simulink model "angle_motor"  (R2021b)
settings: Solver=FixedStepDiscrete  StartTime=0.0  StopTime=inf  FixedStep=0.0005  RelTol=1e-3
model workspace (MAT data in the model file):
  data = 30
  data2 = -30
libraries: simulink x9, IFR_StackLiteDualDrive_SimulinkLib x4
settings Model: Creator=ysl  LastModifiedBy=ysl
settings OptimizationCC: DefaultParameterBehavior=Inlined  EnhancedBackFolding=on  PassReuseOutputArgsAs=Individual arguments  ZeroExternalMemoryAtStartup=off  ZeroInternalMemoryAtStartup=off  OptimizeBlockOrder=speed  DifferentSizesBufferReuse=on  OptimizationCustomize=off  EfficientTunableParamExpr=on
settings DebuggingCC: ParameterTunabilityLossMsg=error
settings SFSimCC: MATLABDynamicMemAlloc=off
settings RTWCC: Description=IFR StackLite-DualDrive Base on stm32f405RGT6  SystemTargetFile=stacklite_dualdrive.tlc  TemplateMakefile=stacklite_dualdrive.tmf  GenerateReport=on
settings CodeAppCC: ForceParamTrailComments=on  IgnoreCustomStorageClasses=off  OperatorAnnotations=on  SimulinkDataObjDesc=on  SFDataObjDesc=on  InsertBlockDesc=on
settings STFCustomTargetCC: TargetLangStandard=C99 (ISO)  MultiwordLength=256  ParMdlRefBuildCompliant=on  CompOptLevelCompliant=on  CombineOutputUpdateFcns=on  ERTCustomFileBanners=on  SupportContinuousTime=off  SupportNonInlinedSFcns=off  RemoveResetFunc=on  MATLABClassNameForMDSCustomization=Simulink.SoftwareTarget.ERTCustomization  CPPClassGenCompliant=on  GRTInterface=off  SystemTargetFile=stacklite_dualdrive.tlc
settings ERTTargetCC: TargetLangStandard=C99 (ISO)  ConcurrentExecutionCompliant=off  ModelStepFunctionPrototypeControlCompliant=off  UseToolchainInfoCompliant=off  InlinedParameterPlacement=NonHierarchical  ERTCustomFileTemplate=example_file_process.tlc

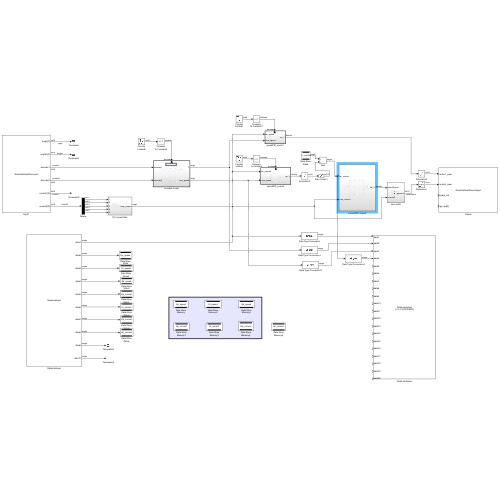
[thumbnail: Simulink's stored preview of the top-level diagram]
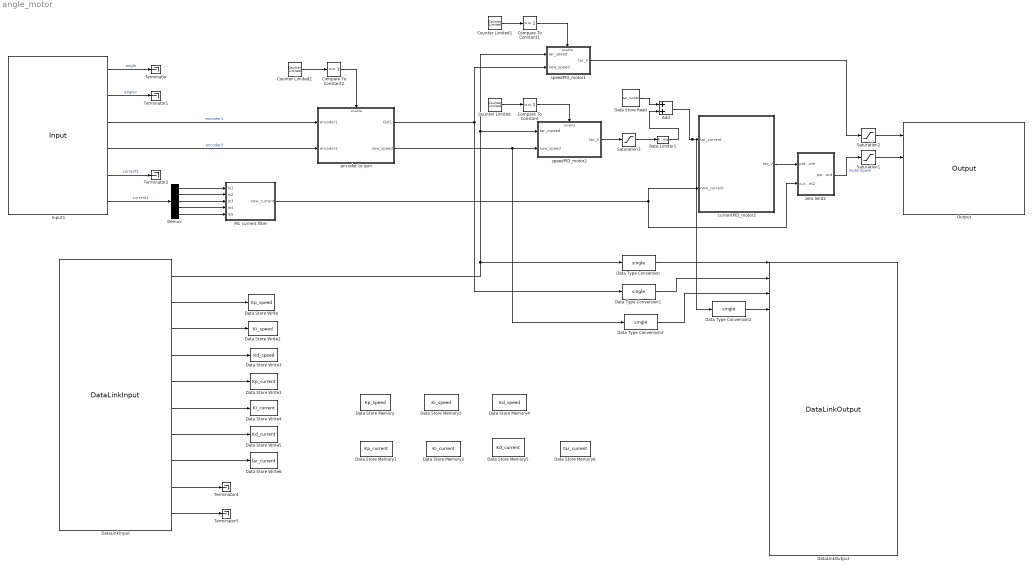
== system angle_motor ==
  Add : Sum
  Compare To Constant : simulink/Logic and Bit Operations/Compare To Constant  relop===  const=1  OutDataTypeStr=boolean
  Compare To Constant1 : simulink/Logic and Bit Operations/Compare To Constant  relop===  const=1  OutDataTypeStr=boolean
  Compare To Constant2 : simulink/Logic and Bit Operations/Compare To Constant  relop===  const=1  OutDataTypeStr=boolean
  Counter Limited : simulink/Sources/Counter Limited  uplimit=1  tsamp=-1
  Counter Limited1 : simulink/Sources/Counter Limited  uplimit=1  tsamp=-1
  Counter Limited2 : simulink/Sources/Counter Limited  uplimit=1  tsamp=-1
  Data Store Memory : DataStoreMemory  DataStoreName=Kp_speed  ReadBeforeWriteMsg=warning  WriteAfterWriteMsg=warning  WriteAfterReadMsg=warning  ShowAdditionalParam=off
  Data Store Memory1 : DataStoreMemory  DataStoreName=Kp_current  ReadBeforeWriteMsg=warning  WriteAfterWriteMsg=warning  WriteAfterReadMsg=warning  ShowAdditionalParam=off
  Data Store Memory2 : DataStoreMemory  DataStoreName=Ki_speed  ReadBeforeWriteMsg=warning  WriteAfterWriteMsg=warning  WriteAfterReadMsg=warning  ShowAdditionalParam=off
  Data Store Memory3 : DataStoreMemory  DataStoreName=Ki_current  ReadBeforeWriteMsg=warning  WriteAfterWriteMsg=warning  WriteAfterReadMsg=warning  ShowAdditionalParam=off
  Data Store Memory4 : DataStoreMemory  DataStoreName=Kd_speed  ReadBeforeWriteMsg=warning  WriteAfterWriteMsg=warning  WriteAfterReadMsg=warning  ShowAdditionalParam=off
  Data Store Memory5 : DataStoreMemory  DataStoreName=Kd_current  ReadBeforeWriteMsg=warning  WriteAfterWriteMsg=warning  WriteAfterReadMsg=warning  ShowAdditionalParam=off
  Data Store Memory6 : DataStoreMemory  DataStoreName=tar_current  ReadBeforeWriteMsg=warning  WriteAfterWriteMsg=warning  WriteAfterReadMsg=warning  ShowAdditionalParam=off
  Data Store Read : DataStoreRead  DataStoreName=tar_current  IndexOptions=Index vector (dialog)  Indices=1  OutputSizes=1
  Data Store Write : DataStoreWrite  DataStoreName=Kp_speed  IndexOptions=Index vector (dialog)  Indices=1  OutputSizes=1
  Data Store Write1 : DataStoreWrite  DataStoreName=Kp_current  IndexOptions=Index vector (dialog)  Indices=1  OutputSizes=1
  Data Store Write2 : DataStoreWrite  DataStoreName=Ki_speed  IndexOptions=Index vector (dialog)  Indices=1  OutputSizes=1
  Data Store Write3 : DataStoreWrite  DataStoreName=Kd_speed  IndexOptions=Index vector (dialog)  Indices=1  OutputSizes=1
  Data Store Write4 : DataStoreWrite  DataStoreName=Ki_current  IndexOptions=Index vector (dialog)  Indices=1  OutputSizes=1
  Data Store Write5 : DataStoreWrite  DataStoreName=Kd_current  IndexOptions=Index vector (dialog)  Indices=1  OutputSizes=1
  Data Store Write6 : DataStoreWrite  DataStoreName=tar_current  IndexOptions=Index vector (dialog)  Indices=1  OutputSizes=1
  Data Type Conversion{,1..3} (4 alike) : DataTypeConversion  OutDataTypeStr=single
  DataLinkInput : IFR_StackLiteDualDrive_SimulinkLib/DataLinkInput
      settings: SourceProductName=IFR_StackLiteDualDrive_SimulinkLib_V1.0
  DataLinkOutput : IFR_StackLiteDualDrive_SimulinkLib/DataLinkOutput  id='BalanceUnname'  key='IFR00'
      settings: SourceProductName=IFR_StackLiteDualDrive_SimulinkLib_V1.0
  Demux : Demux  Outputs=5
  Input1 : IFR_StackLiteDualDrive_SimulinkLib/Input  Priority=0
      settings: SourceProductName=IFR_StackLiteDualDrive_SimulinkLib_V1.0
  M1 current filter : Subsystem
  Output : IFR_StackLiteDualDrive_SimulinkLib/Output  Priority=255
      settings: SourceProductName=IFR_StackLiteDualDrive_SimulinkLib_V1.0
  Rate Limiter1 : RateLimiter  RisingSlewLimit=10000  FallingSlewLimit=-10000  SampleTimeMode=inherited
  Saturation1 : Saturate  UpperLimit=4200  LowerLimit=-4200  OutDataTypeStr=int16
  Saturation2 : Saturate  UpperLimit=4200  LowerLimit=-4200  OutDataTypeStr=int16
  Saturation3 : Saturate  UpperLimit=2048  LowerLimit=-2048  OutDataTypeStr=int16
  Terminator{,1..2,4..5} (5 alike) : Terminator
  currentPID_motor2 : Subsystem
  encoder to rpm : Subsystem
  speedPID_motor1 : Subsystem
  speedPID_motor2 : Subsystem
  zero limit2 : Subsystem
  wires:
  Input1/6 -> Demux/1  "current1"
  Demux/1 -> M1 current filter/1(In1)
  Demux/2 -> M1 current filter/2(In2)
  Demux/3 -> M1 current filter/3(In3)
  Demux/4 -> M1 current filter/4(In4)
  Demux/5 -> M1 current filter/5(In5)
  DataLinkInput/2 -> Data Store Write/1
  DataLinkInput/3 -> Data Store Write2/1
  DataLinkInput/4 -> Data Store Write3/1
  DataLinkInput/5 -> Data Store Write1/1
  DataLinkInput/6 -> Data Store Write4/1
  DataLinkInput/7 -> Data Store Write5/1
  Input1/1 -> Terminator/1  "angle"
  Input1/2 -> Terminator1/1  "anglev"
  DataLinkInput/9 -> Terminator4/1
  DataLinkInput/10 -> Terminator5/1
  Data Type Conversion/1 -> DataLinkOutput/1
  Data Type Conversion1/1 -> DataLinkOutput/2
  Input1/5 -> Terminator2/1  "current1"
  speedPID_motor2/1(tar_V) -> Saturation3/1
  Counter Limited/1 -> Compare To Constant/1
  Compare To Constant/1 -> speedPID_motor2/Enable
  DataLinkInput/1 -> speedPID_motor2/1(tar_cspeed), speedPID_motor1/1(tar_speed), Data Type Conversion/1
  speedPID_motor1/1(tar_V) -> Saturation2/1
  Counter Limited1/1 -> Compare To Constant1/1
  Compare To Constant1/1 -> speedPID_motor1/Enable
  Saturation3/1 -> Rate Limiter1/1
  M1 current filter/1(now_current) -> zero limit2/2(current2), currentPID_motor2/2(now_current)
  Saturation1/1 -> Output/2
  encoder to rpm/1(Out1) -> Data Type Conversion1/1, speedPID_motor1/2(now_speed)
  Input1/3 -> encoder to rpm/1(encoder1)  "encoder1"
  Input1/4 -> encoder to rpm/2(encoder2)  "encoder2"
  Counter Limited2/1 -> Compare To Constant2/1
  Compare To Constant2/1 -> encoder to rpm/Enable
  encoder to rpm/2(now_speed) -> Data Type Conversion3/1, speedPID_motor2/2(now_speed)
  currentPID_motor2/1(tar_V) -> zero limit2/1(pidout2pwm)
  zero limit2/1(pwmout) -> Saturation1/1  "motor2pwm"
  Saturation2/1 -> Output/1
  Data Type Conversion3/1 -> DataLinkOutput/3
  DataLinkInput/8 -> Data Store Write6/1
  Data Store Read/1 -> Add/1
  Rate Limiter1/1 -> Add/2
  Add/1 -> currentPID_motor2/1(tar_current), Data Type Conversion2/1
  Data Type Conversion2/1 -> DataLinkOutput/4

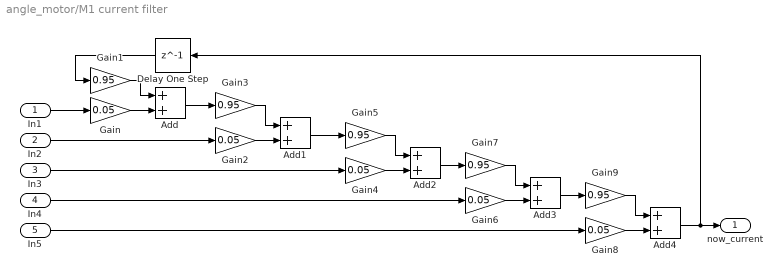
== system angle_motor/M1 current filter ==
  In1 : Inport
  In2 : Inport  Port=2
  In3 : Inport  Port=3
  In4 : Inport  Port=4
  In5 : Inport  Port=5
  Add{,1..4} (5 alike) : Sum
  Delay One Step : Delay  DelayLength=1
  Gain{,2,4,6,8} (5 alike) : Gain  Gain=0.05  OutDataTypeStr=single
  Gain{1,3,5,7,9} (5 alike) : Gain  Gain=0.95  OutDataTypeStr=single
  now_current : Outport
  wires:
  Add4/1 -> now_current/1, Delay One Step/1
  In5/1 -> Gain8/1
  Add3/1 -> Gain9/1
  Gain9/1 -> Add4/1
  Gain8/1 -> Add4/2
  In4/1 -> Gain6/1
  Add2/1 -> Gain7/1
  Gain7/1 -> Add3/1
  Gain6/1 -> Add3/2
  In3/1 -> Gain4/1
  Add1/1 -> Gain5/1
  Gain5/1 -> Add2/1
  Gain4/1 -> Add2/2
  In2/1 -> Gain2/1
  Gain3/1 -> Add1/1
  Gain2/1 -> Add1/2
  Add/1 -> Gain3/1
  Gain1/1 -> Add/1
  Delay One Step/1 -> Gain1/1
  Gain/1 -> Add/2
  In1/1 -> Gain/1

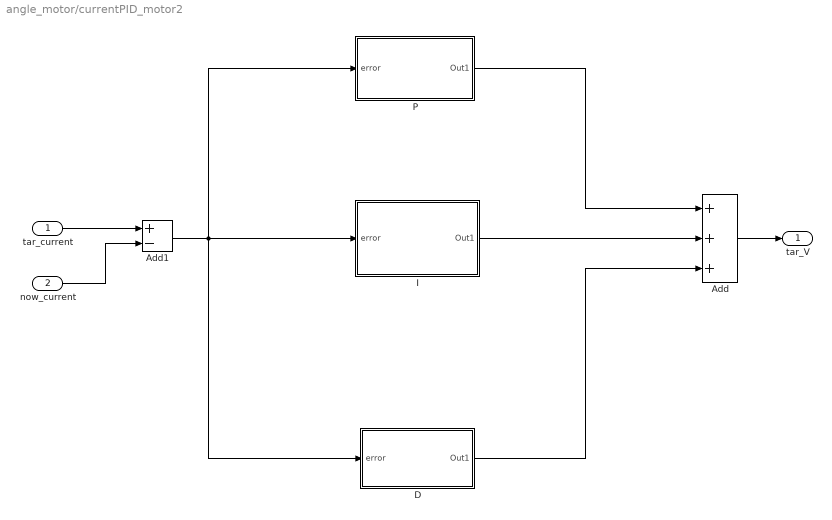
== system angle_motor/currentPID_motor2 ==
  tar_current : Inport
  now_current : Inport  Port=2
  Add : Sum  Inputs=+++  OutDataTypeStr=double
  Add1 : Sum  Inputs=+-
  D : Subsystem
  I : Subsystem
  P : Subsystem
  tar_V : Outport
  wires:
  now_current/1 -> Add1/2
  Add/1 -> tar_V/1
  tar_current/1 -> Add1/1
  Add1/1 -> D/1(error), I/1(error), P/1(error)
  P/1(Out1) -> Add/1
  I/1(Out1) -> Add/2
  D/1(Out1) -> Add/3

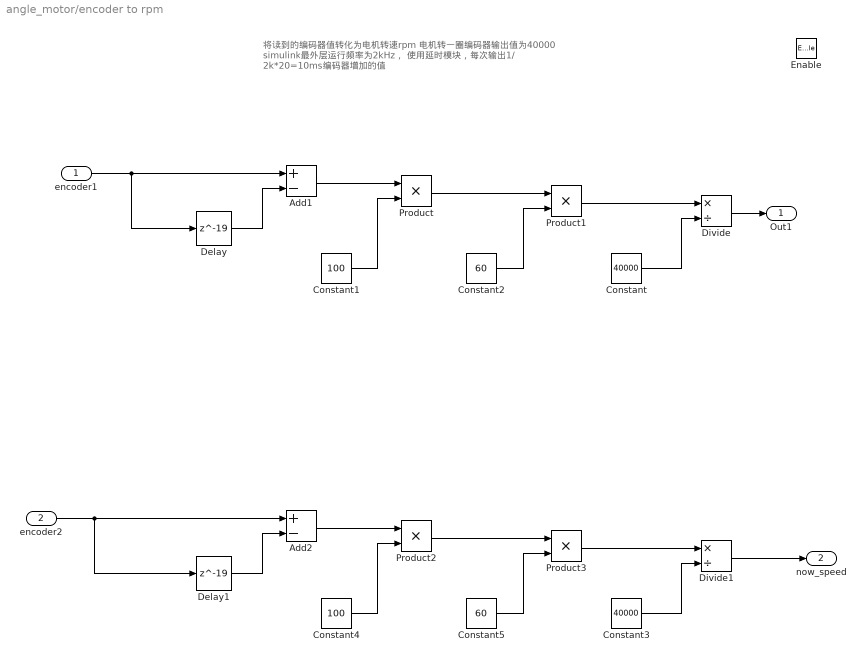
== system angle_motor/encoder to rpm ==
  note: 将读到的编码器值转化为电机转速rpm
      | 电机转一圈编码器输出值为40000
      | simulink最外层运行频率为2kHz，
      | 使用延时模块，每次输出1/ 2k*20=10ms编码器增加的值
  encoder1 : Inport
  encoder2 : Inport  Port=2
  Enable : EnablePort
  Add1 : Sum  Inputs=+-
  Add2 : Sum  Inputs=+-
  Constant : Constant  Value=40000  OutDataTypeStr=single
  Constant1 : Constant  Value=100  OutDataTypeStr=single
  Constant2 : Constant  Value=60  OutDataTypeStr=single
  Constant3 : Constant  Value=40000  OutDataTypeStr=single
  Constant4 : Constant  Value=100  OutDataTypeStr=single
  Constant5 : Constant  Value=60  OutDataTypeStr=single
  Delay : Delay  DelayLength=19
  Delay1 : Delay  DelayLength=19
  Divide : Product  Inputs=*/  OutDataTypeStr=single
  Divide1 : Product  Inputs=*/  OutDataTypeStr=single
  Product{,1..3} (4 alike) : Product  OutDataTypeStr=single
  Out1 : Outport
  now_speed : Outport  Port=2
  wires:
  Product1/1 -> Divide/1
  Product/1 -> Product1/1
  Constant/1 -> Divide/2
  encoder1/1 -> Add1/1, Delay/1
  Add2/1 -> Product2/1
  Delay1/1 -> Add2/2
  encoder2/1 -> Add2/1, Delay1/1
  Constant1/1 -> Product/2
  Add1/1 -> Product/1
  Constant2/1 -> Product1/2
  Delay/1 -> Add1/2
  Divide1/1 -> now_speed/1
  Product2/1 -> Product3/1
  Constant4/1 -> Product2/2
  Product3/1 -> Divide1/1
  Constant5/1 -> Product3/2
  Divide/1 -> Out1/1
  Constant3/1 -> Divide1/2

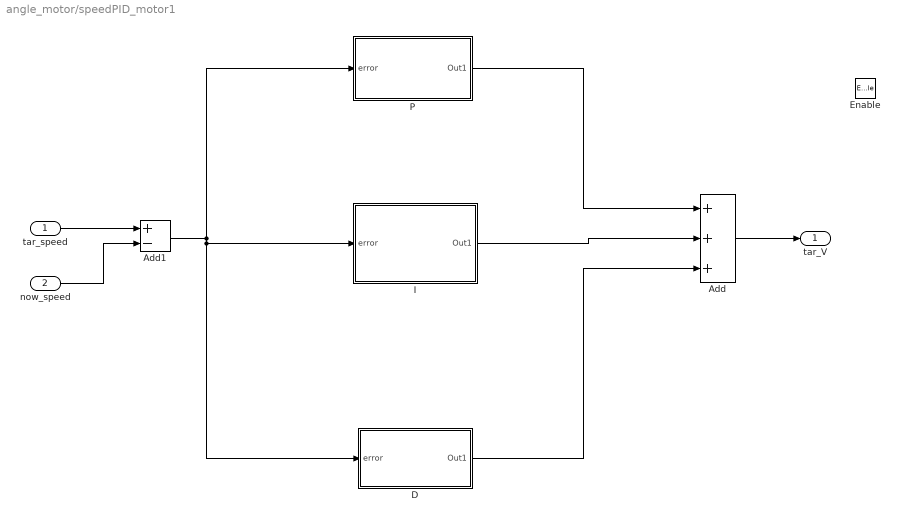
== system angle_motor/speedPID_motor1 ==
  tar_speed : Inport
  now_speed : Inport  Port=2
  Enable : EnablePort
  Add : Sum  Inputs=+++  OutDataTypeStr=double
  Add1 : Sum  Inputs=+-
  D : Subsystem
  I : Subsystem
  P : Subsystem
  tar_V : Outport
  wires:
  D/1(Out1) -> Add/3
  tar_speed/1 -> Add1/1
  P/1(Out1) -> Add/1
  Add/1 -> tar_V/1
  Add1/1 -> D/1(error), I/1(error), P/1(error)
  now_speed/1 -> Add1/2
  I/1(Out1) -> Add/2

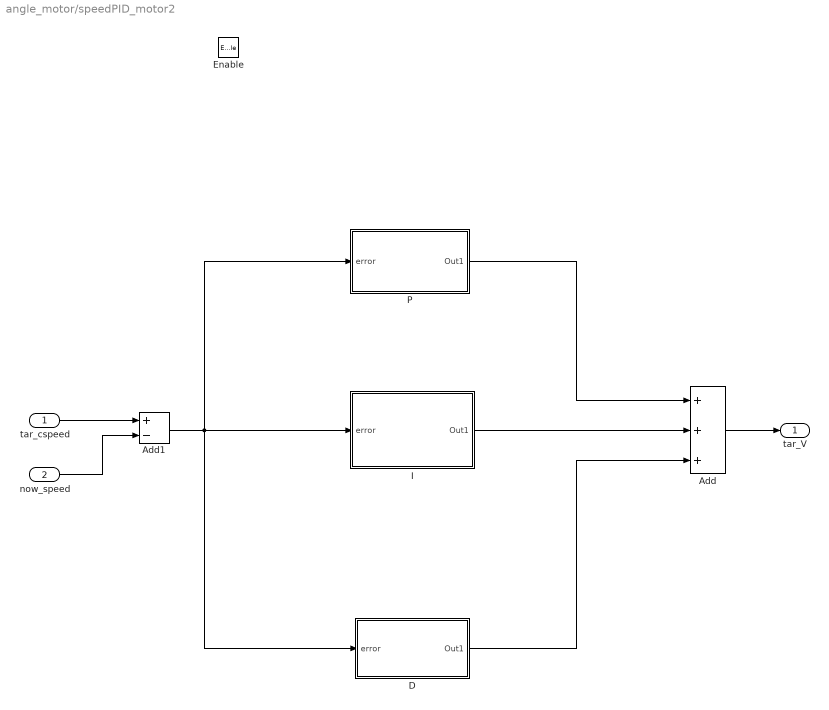
== system angle_motor/speedPID_motor2 ==
  tar_cspeed : Inport
  now_speed : Inport  Port=2
  Enable : EnablePort
  Add : Sum  Inputs=+++  OutDataTypeStr=double
  Add1 : Sum  Inputs=+-
  D : Subsystem
  I : Subsystem
  P : Subsystem
  tar_V : Outport
  wires:
  Add/1 -> tar_V/1
  now_speed/1 -> Add1/2
  I/1(Out1) -> Add/2
  P/1(Out1) -> Add/1
  Add1/1 -> D/1(error), I/1(error), P/1(error)
  D/1(Out1) -> Add/3
  tar_cspeed/1 -> Add1/1

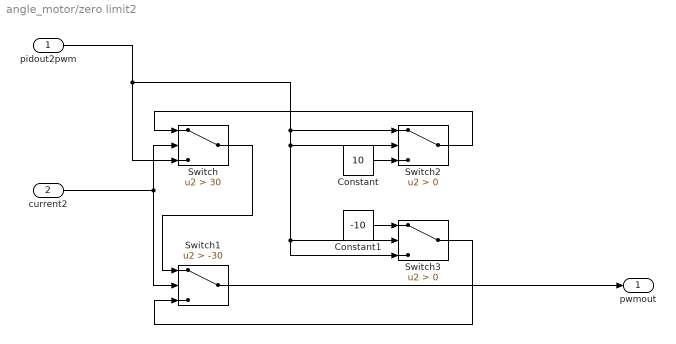
== system angle_motor/zero limit2 ==
  pidout2pwm : Inport
  current2 : Inport  Port=2
  Constant : Constant  Value=10  OutDataTypeStr=int16
  Constant1 : Constant  Value=-10  OutDataTypeStr=int16
  Switch : Switch  Criteria=u2 > Threshold  Threshold=30  OutDataTypeStr=int16
  Switch1 : Switch  Criteria=u2 > Threshold  Threshold=-30  OutDataTypeStr=int16
  Switch2 : Switch  Criteria=u2 > Threshold  OutDataTypeStr=int16
  Switch3 : Switch  Criteria=u2 > Threshold  OutDataTypeStr=int16
  pwmout : Outport
  wires:
  Switch1/1 -> pwmout/1
  Switch2/1 -> Switch/1
  Switch3/1 -> Switch1/3
  Switch/1 -> Switch1/1
  Constant/1 -> Switch2/3
  pidout2pwm/1 -> Switch2/2, Switch3/2, Switch3/3, Switch2/1, Switch/3
  current2/1 -> Switch1/2, Switch/2
  Constant1/1 -> Switch3/1

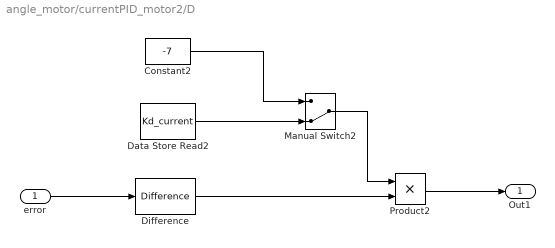
== system angle_motor/currentPID_motor2/D ==
  error : Inport
  Constant2 : Constant  Value=-7
  Data Store Read2 : DataStoreRead  DataStoreName=Kd_current  IndexOptions=Index vector (dialog)  Indices=1  OutputSizes=1
  Difference : simulink/Discrete/Difference  ICPrevInput=0.0  OutMin=[]  OutMax=[]  OutDataType=fixdt(1, 16)  OutScaling=2^-10  DoSatur=off
  Manual Switch2 : ManualSwitch  CurrentSetting=0
  Product2 : Product
  Out1 : Outport
  wires:
  Difference/1 -> Product2/2
  Product2/1 -> Out1/1
  Data Store Read2/1 -> Manual Switch2/2
  Manual Switch2/1 -> Product2/1
  Constant2/1 -> Manual Switch2/1
  error/1 -> Difference/1

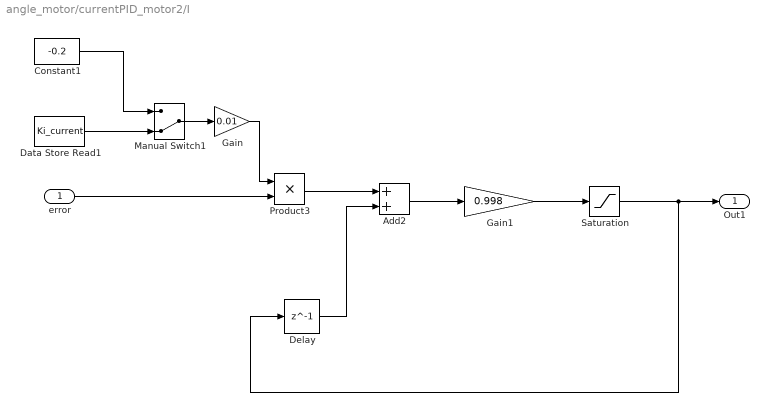
== system angle_motor/currentPID_motor2/I ==
  error : Inport
  Add2 : Sum
  Constant1 : Constant  Value=-0.2
  Data Store Read1 : DataStoreRead  DataStoreName=Ki_current  IndexOptions=Index vector (dialog)  Indices=1  OutputSizes=1
  Delay : Delay  DelayLength=1
  Gain : Gain  Gain=0.01
  Gain1 : Gain  Gain=0.998
  Manual Switch1 : ManualSwitch  CurrentSetting=0
  Product3 : Product  OutDataTypeStr=single
  Saturation : Saturate  UpperLimit=2000  LowerLimit=-2000
  Out1 : Outport
  wires:
  Delay/1 -> Add2/2
  Gain/1 -> Product3/1
  Add2/1 -> Gain1/1
  Constant1/1 -> Manual Switch1/1
  Manual Switch1/1 -> Gain/1
  Data Store Read1/1 -> Manual Switch1/2
  Product3/1 -> Add2/1
  error/1 -> Product3/2
  Gain1/1 -> Saturation/1
  Saturation/1 -> Delay/1, Out1/1

== system angle_motor/currentPID_motor2/P ==
  error : Inport
  Constant : Constant  Value=-2
  Data Store Read : DataStoreRead  DataStoreName=Kp_current  IndexOptions=Index vector (dialog)  Indices=1  OutputSizes=1
  Manual Switch : ManualSwitch  CurrentSetting=0
  Product : Product
  Out1 : Outport
  wires:
  error/1 -> Product/2
  Manual Switch/1 -> Product/1
  Data Store Read/1 -> Manual Switch/2
  Constant/1 -> Manual Switch/1
  Product/1 -> Out1/1

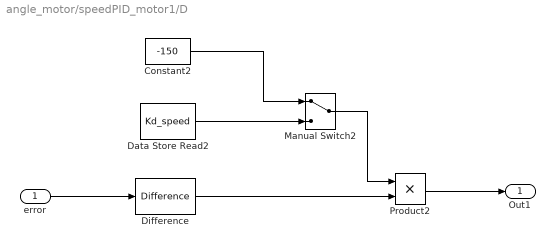
== system angle_motor/speedPID_motor1/D ==
  error : Inport
  Constant2 : Constant  Value=-150
  Data Store Read2 : DataStoreRead  DataStoreName=Kd_speed  IndexOptions=Index vector (dialog)  Indices=1  OutputSizes=1
  Difference : simulink/Discrete/Difference  ICPrevInput=0.0  OutMin=[]  OutMax=[]  OutDataType=fixdt(1, 16)  OutScaling=2^-10  DoSatur=off
  Manual Switch2 : ManualSwitch
  Product2 : Product
  Out1 : Outport
  wires:
  Difference/1 -> Product2/2
  Product2/1 -> Out1/1
  Data Store Read2/1 -> Manual Switch2/2
  Manual Switch2/1 -> Product2/1
  Constant2/1 -> Manual Switch2/1
  error/1 -> Difference/1

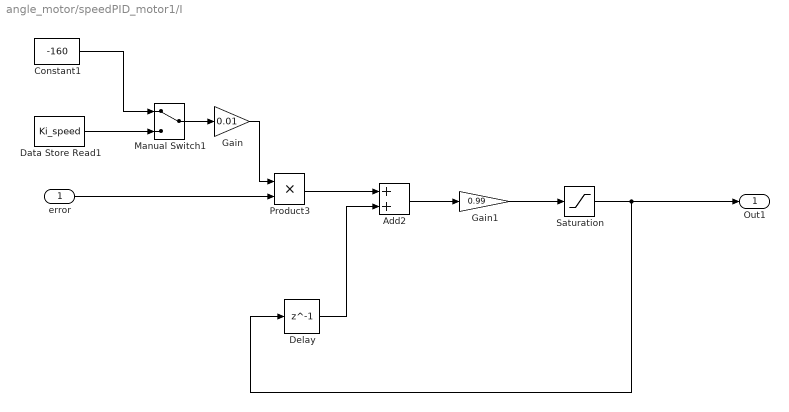
== system angle_motor/speedPID_motor1/I ==
  error : Inport
  Add2 : Sum
  Constant1 : Constant  Value=-160
  Data Store Read1 : DataStoreRead  DataStoreName=Ki_speed  IndexOptions=Index vector (dialog)  Indices=1  OutputSizes=1
  Delay : Delay  DelayLength=1
  Gain : Gain  Gain=0.01
  Gain1 : Gain  Gain=0.99
  Manual Switch1 : ManualSwitch
  Product3 : Product  OutDataTypeStr=single
  Saturation : Saturate  UpperLimit=600  LowerLimit=-600
  Out1 : Outport
  wires:
  Delay/1 -> Add2/2
  Gain/1 -> Product3/1
  Add2/1 -> Gain1/1
  Constant1/1 -> Manual Switch1/1
  Manual Switch1/1 -> Gain/1
  Data Store Read1/1 -> Manual Switch1/2
  Gain1/1 -> Saturation/1
  Product3/1 -> Add2/1
  error/1 -> Product3/2
  Saturation/1 -> Out1/1, Delay/1

== system angle_motor/speedPID_motor1/P ==
  error : Inport
  Constant : Constant  Value=-40
  Data Store Read : DataStoreRead  DataStoreName=Kp_speed  IndexOptions=Index vector (dialog)  Indices=1  OutputSizes=1
  Manual Switch : ManualSwitch
  Product : Product
  Out1 : Outport
  wires:
  error/1 -> Product/2
  Manual Switch/1 -> Product/1
  Data Store Read/1 -> Manual Switch/2
  Constant/1 -> Manual Switch/1
  Product/1 -> Out1/1

== system angle_motor/speedPID_motor2/D ==
  error : Inport
  Constant2 : Constant  Value=55
  Data Store Read2 : DataStoreRead  DataStoreName=Kd_speed  IndexOptions=Index vector (dialog)  Indices=1  OutputSizes=1
  Difference : simulink/Discrete/Difference  ICPrevInput=0.0  OutMin=[]  OutMax=[]  OutDataType=fixdt(1, 16)  OutScaling=2^-10  DoSatur=off
  Manual Switch2 : ManualSwitch  CurrentSetting=0
  Product2 : Product
  Out1 : Outport
  wires:
  Difference/1 -> Product2/2
  Product2/1 -> Out1/1
  Data Store Read2/1 -> Manual Switch2/2
  Manual Switch2/1 -> Product2/1
  Constant2/1 -> Manual Switch2/1
  error/1 -> Difference/1

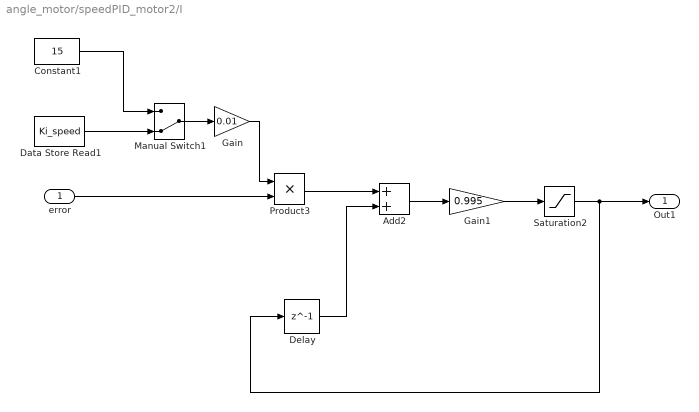
== system angle_motor/speedPID_motor2/I ==
  error : Inport
  Add2 : Sum
  Constant1 : Constant  Value=15
  Data Store Read1 : DataStoreRead  DataStoreName=Ki_speed  IndexOptions=Index vector (dialog)  Indices=1  OutputSizes=1
  Delay : Delay  DelayLength=1
  Gain : Gain  Gain=0.01
  Gain1 : Gain  Gain=0.995
  Manual Switch1 : ManualSwitch  CurrentSetting=0
  Product3 : Product  OutDataTypeStr=single
  Saturation2 : Saturate  UpperLimit=1500  LowerLimit=-1500
  Out1 : Outport
  wires:
  Delay/1 -> Add2/2
  Gain/1 -> Product3/1
  Add2/1 -> Gain1/1
  Constant1/1 -> Manual Switch1/1
  Manual Switch1/1 -> Gain/1
  Data Store Read1/1 -> Manual Switch1/2
  Gain1/1 -> Saturation2/1
  Product3/1 -> Add2/1
  error/1 -> Product3/2
  Saturation2/1 -> Out1/1, Delay/1

== system angle_motor/speedPID_motor2/P ==
  error : Inport
  Constant : Constant  Value=1.5
  Data Store Read : DataStoreRead  DataStoreName=Kp_speed  IndexOptions=Index vector (dialog)  Indices=1  OutputSizes=1
  Manual Switch : ManualSwitch  CurrentSetting=0
  Product : Product
  Out1 : Outport
  wires:
  error/1 -> Product/2
  Manual Switch/1 -> Product/1
  Data Store Read/1 -> Manual Switch/2
  Constant/1 -> Manual Switch/1
  Product/1 -> Out1/1
